simulink model "estimator"  (R2024a)
settings: Solver=VariableStepAuto  StartTime=0.0  StopTime=10.0  RelTol=1e-3
values from neighbouring files (symbols this model uses):
  J = 0.02    [ControlSystemFinal_ChoiChiHyuk.m]
  K = acker(A,B,desired_poles)    [ControlSystemFinal_ChoiChiHyuk.m]
  Kb = 0.015    [ControlSystemFinal_ChoiChiHyuk.m]
  Kf = 0.2    [ControlSystemFinal_ChoiChiHyuk.m]
  Km = 0.015    [ControlSystemFinal_ChoiChiHyuk.m]
  L = 0.5    [ControlSystemFinal_ChoiChiHyuk.m]
  L_esti = acker(A,B,desired_error)    [ControlSystemFinal_ChoiChiHyuk.m]
  Nb = Nu+K*Nx    [ControlSystemFinal_ChoiChiHyuk.m]
  R = 2.0    (= 2)    [ControlSystemFinal_ChoiChiHyuk.m]
settings Model: Creator=CHI  LastModifiedBy=kevin

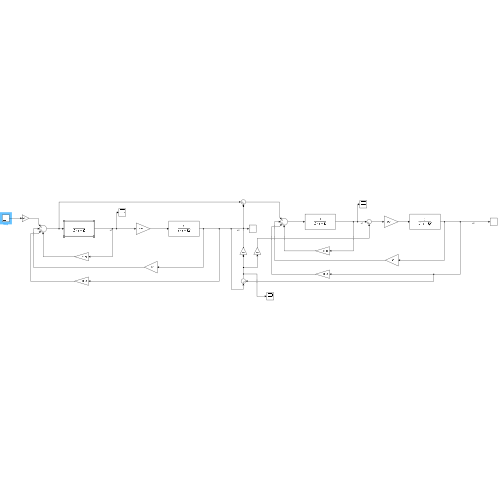
[thumbnail: Simulink's stored preview of the top-level diagram]
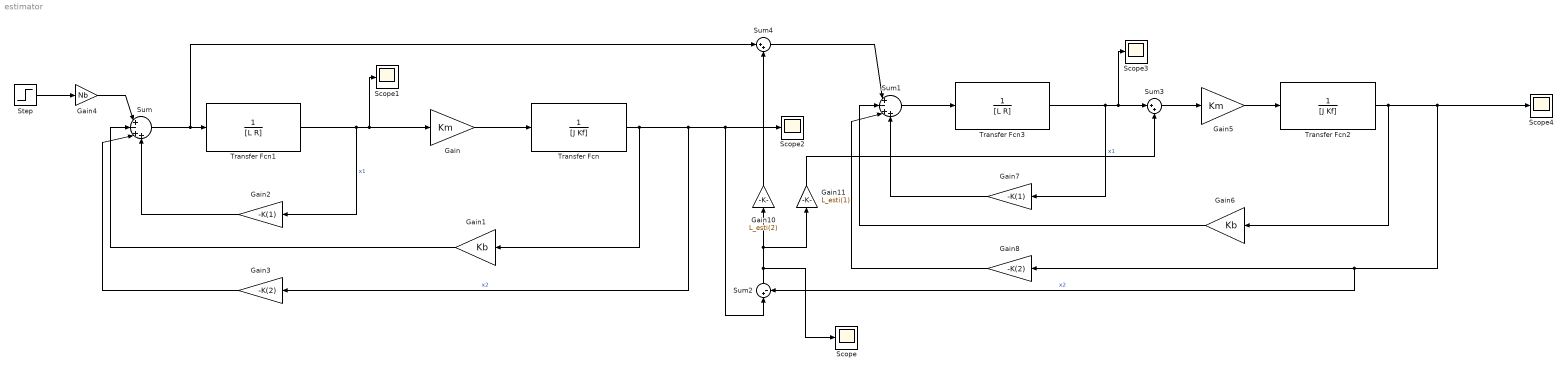
== system estimator ==
  Gain : Gain  Gain=Km
  Gain1 : Gain  Gain=Kb
  Gain10 : Gain  Gain=L_esti(2)
  Gain11 : Gain  Gain=L_esti(1)
  Gain2 : Gain  Gain=-K(1)
  Gain3 : Gain  Gain=-K(2)
  Gain4 : Gain  Gain=Nb
  Gain5 : Gain  Gain=Km
  Gain6 : Gain  Gain=Kb
  Gain7 : Gain  Gain=-K(1)
  Gain8 : Gain  Gain=-K(2)
  Scope{,1..4} (5 alike) : Scope
  Step : Step  SampleTime=0
  Sum : Sum  Inputs=|+-++
  Sum1 : Sum  Inputs=|+-++
  Sum2 : Sum  Inputs=|+-
  Sum3 : Sum  Inputs=|++
  Sum4 : Sum  Inputs=|++
  Transfer Fcn : TransferFcn  Denominator=[J Kf]
  Transfer Fcn1 : TransferFcn  Denominator=[L R]
  Transfer Fcn2 : TransferFcn  Denominator=[J Kf]
  Transfer Fcn3 : TransferFcn  Denominator=[L R]
  wires:
  Sum/1 -> Sum4/1, Transfer Fcn1/1
  Transfer Fcn1/1 -> Gain2/1, Scope1/1, Gain/1  "x1"
  Gain/1 -> Transfer Fcn/1
  Gain1/1 -> Sum/2
  Gain3/1 -> Sum/3
  Transfer Fcn/1 -> Gain3/1, Sum2/1, Scope2/1, Gain1/1  "x2"
  Gain2/1 -> Sum/4
  Gain4/1 -> Sum/1
  Sum1/1 -> Transfer Fcn3/1
  Transfer Fcn3/1 -> Gain7/1, Sum3/1, Scope3/1  "x1"
  Gain5/1 -> Transfer Fcn2/1
  Gain6/1 -> Sum1/2
  Gain8/1 -> Sum1/3
  Transfer Fcn2/1 -> Sum2/2, Gain8/1, Scope4/1, Gain6/1  "x2"
  Gain7/1 -> Sum1/4
  Step/1 -> Gain4/1
  Sum3/1 -> Gain5/1
  Sum2/1 -> Scope/1, Gain11/1, Gain10/1
  Gain11/1 -> Sum3/2
  Gain10/1 -> Sum4/2
  Sum4/1 -> Sum1/1
